simulink model "SlidingModeControl"  (R2018a)
settings: Solver=ode45  StartTime=0.0  StopTime=400  RelTol=1e-3  EnableMultiTasking=on
undefined symbols (not defined in the file or in its folder): sigbuilder_block
libraries: arduino_io_lib x4
settings Model: Creator=Gabriel  LastModifiedBy=Aluno
settings DataIOCC: LimitDataPoints=on  SaveFormat=Array
settings OptimizationCC: LifeSpan=inf
settings DebuggingCC: UnderspecifiedInitializationDetection=Classic  MergeDetectMultiDrivingBlocksExec=none  SolverPrmCheckMsg=warning  StateNameClashWarn=warning  SFUnexpectedBacktrackingDiag=warning  SFNoUnconditionalDefaultTransitionDiag=warning  SFExecutionAtInitializationDiag=none
settings HardwareCC: ProdBitPerPointer=32  ProdBitPerSizeT=32  ProdBitPerPtrDiffT=32  ProdLargestAtomicFloat=None  ProdIntDivRoundTo=Undefined  ProdEndianess=Unspecified  ProdWordSize=32  ProdHWDeviceType=32-bit Generic
settings ModelReferenceCC: PropagateSignalLabelsOutOfModel=off
settings CodeAppCC: StateflowObjectComments=on
settings GRTTargetCC: TargetLangStandard=C89/C90 (ANSI)  GeneratePreprocessorConditionals=Disable all
settings ConfigComp: CovMetricSettings=dw  CovHtmlReporting=on  CovSaveCumulativeToWorkspaceVar=on  CovSaveSingleToWorkspaceVar=on  CovExternalEMLEnable=off

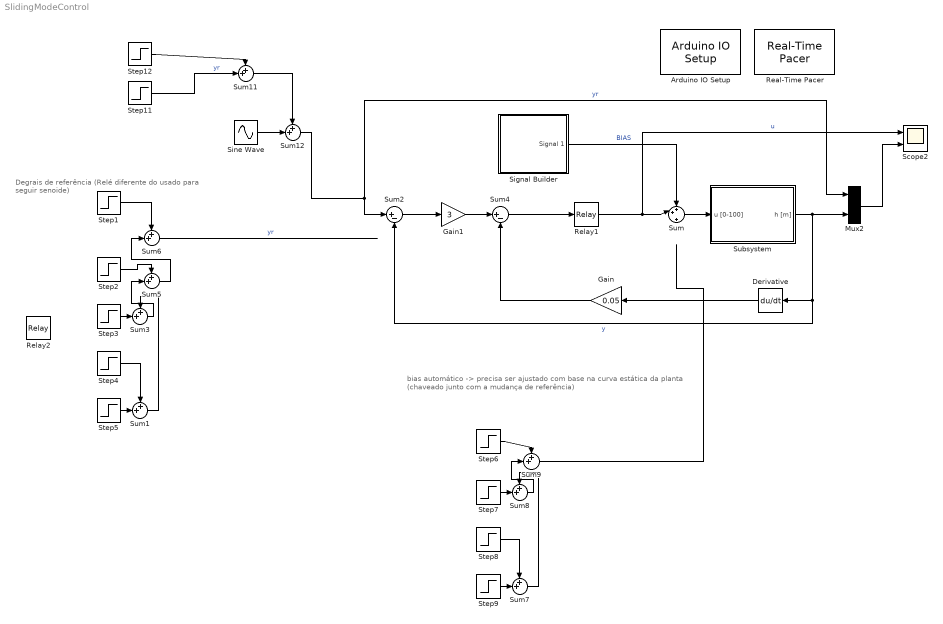
== system SlidingModeControl ==
  note: Degrais de
      | referência
      |
      |
      |
      |
      |
      | (Relé diferente
      | do usado
      | para seguir
      | senoide)
  note: bias automático
      | -> precisa ser ajustado com base na curva estática da planta
      | (chaveado junto com a mudança de referência)
  Arduino IO Setup : arduino_io_lib/Arduino IO Setup  Priority=3  arduinoVar=Temporary arduino variable: Arduino1  workspaceVarName=a  comPort=COM7
  Derivative : Derivative
  Gain : Gain  Gain=0.05
  Gain1 : Gain  Gain=3
  Mux2 : Mux  Inputs=2
  Real-Time Pacer : arduino_io_lib/Real-Time Pacer  simTimePerRealTime=1
  Relay1 : Relay  OffSwitchValue=-eps  OnOutputValue=3
  Relay2 : Relay  OffSwitchValue=-eps  OnOutputValue=1.5
  Scope2 : Scope  NumInputPorts=2
  Signal Builder : Subsystem  Tag=STV Subsys  LoadFcn=sigbuilder_block('load');  StartFcn=sigbuilder_block('start');  StopFcn=sigbuilder_block('stop');  ClipboardFcn=sigbuilder_block('clipboard');  mask(Sigbuilder block){tuvar=[0:10]}
      mask help: Simulink:masks:SigbuilderBlock_MD
      mask init:
      | if ~strcmp(get_param(bdroot(gcbh),'SimulationStatus'),'stopped') tuvar = sigbuilder_block('maskInit'); end
      settings: CopyFcn=sigbuilder_block('copy');  DeleteFcn=sigbuilder_block('delete');  ModelCloseFcn=sigbuilder_block('modelClose');  PreSaveFcn=sigbuilder_block('preSave');  PauseFcn=sigbuilder_block('pause');  ContinueFcn=sigbuilder_block('continue');  NameChangeFcn=sigbuilder_block('namechange');  OpenFcn=sigbuilder_block('open',[6 30 1188 546.75 ]);  CloseFcn=sigbuilder_block('close');
      mask Display: plot(0, 0, 100, 100,[2, 2, 32, 32, 2], [68, 8, 8, 68, 68],[32, 2], [38, 38], [32, 19, 2],[53, 60, 44], [32, 17, 17, 2],[16, 16, 31, 31]);txt = getActiveGroup(gcbh);text(2, 100, txt,'verticalAlignment', 'top');
  Sine Wave : Sin  Amplitude=0.05  Frequency=0.2  SampleTime=0
  Step1 : Step  Time=25  Before=0.6  After=0.55  SampleTime=0
  Step11 : Step  Time=25  Before=0.7  After=0.7  SampleTime=0
  Step12 : Step  Time=0  After=-0.2  SampleTime=0
  Step2 : Step  Time=50  After=0.05  SampleTime=0
  Step3 : Step  Time=75  After=-0.05  SampleTime=0
  Step4 : Step  Time=100  After=-0.05  SampleTime=0
  Step5 : Step  Time=125  After=+0.1  SampleTime=0
  Step6 : Step  Time=50  After=1.5  SampleTime=0
  Step7 : Step  Time=75  After=-1.5  SampleTime=0
  Step8 : Step  Time=100  After=0  SampleTime=0
  Step9 : Step  Time=125  SampleTime=0
  Subsystem : Subsystem
  Sum : Sum  Inputs=++|+
  Sum{1,3,5..9,11..12} (9 alike) : Sum  Inputs=++|
  Sum2 : Sum  Inputs=|+-
  Sum4 : Sum  Inputs=|+-
  wires:
  Subsystem/1(h [m]) -> Mux2/2, Sum2/2, Derivative/1  "y"
  Sum/1 -> Subsystem/1(u [0-100])
  Signal Builder/1(Signal 1) -> Sum/1  "BIAS"
  Gain1/1 -> Sum4/1
  Gain/1 -> Sum4/2
  Sum2/1 -> Gain1/1
  Relay1/1 -> Scope2/1, Sum/2  "u"
  Sum4/1 -> Relay1/1
  Derivative/1 -> Gain/1
  Mux2/1 -> Scope2/2
  Step5/1 -> Sum1/2
  Step4/1 -> Sum1/1
  Sum1/1 -> Sum3/1
  Step3/1 -> Sum3/2
  Sum3/1 -> Sum5/2
  Step2/1 -> Sum5/1
  Step1/1 -> Sum6/1
  Sum5/1 -> Sum6/2
  Sum7/1 -> Sum8/1
  Step8/1 -> Sum7/1
  Sum8/1 -> Sum9/2
  Step7/1 -> Sum8/2
  Step9/1 -> Sum7/2
  Step6/1 -> Sum9/1
  Sum12/1 -> Mux2/1, Sum2/1  "yr"
  Step12/1 -> Sum11/1
  Step11/1 -> Sum11/2  "yr"
  Sum11/1 -> Sum12/1
  Sine Wave/1 -> Sum12/2
  Sum9/1 -> ?
  Sum6/1 -> ?  "yr"

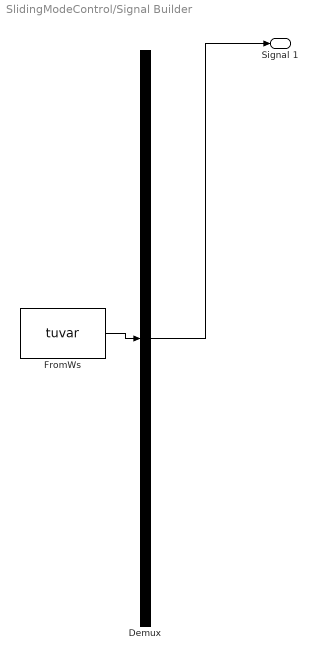
== system SlidingModeControl/Signal Builder ==
  Demux : Demux  Tag=STV Demux  Outputs=1
  FromWs : FromWorkspace  Tag=STV FromWs  VariableName=tuvar  SampleTime=0
      SigBuilderData=|
      | common.afterFinalStr = 'Extrapolate'
      | common.sampleTime = 0
      | dataSet.timeRange = [0 50]
      | dataSet.name = 'Group 1'
      | sbobj.Groups.Name = 'Group 1'
      | sbobj.Groups.Signals.Name = 'Signal 1'
      | sbobj.Groups.Signals.XData = [0 1 1 1.4 1.4 50]
      | sbobj.Groups.Signals.YData = [0 0 74.2 74.2 38.5 38.5]
      | sbobj.Groups.TimeRange = [0 50]
  Signal 1 : Outport  Tag=STV Outport
  wires:
  Demux/1 -> Signal 1/1
  FromWs/1 -> Demux/1

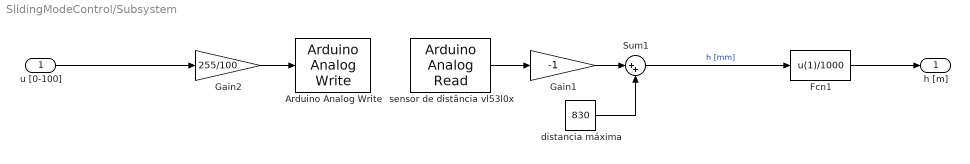
== system SlidingModeControl/Subsystem ==
  u [0-100] : Inport
  Arduino Analog Write : arduino_io_lib/Arduino Analog Write  arduinoVar=Temporary arduino variable: Arduino1  arduinoPin=5  T=0.2
  Fcn1 : Fcn  Expr=u(1)/1000
  Gain1 : Gain  Gain=-1
  Gain2 : Gain  Gain=255/100
  Sum1 : Sum  Inputs=|++
  distancia máxima : Constant  Value=830
  "sensor de distância vl53l0x " : arduino_io_lib/Arduino Analog Read  arduinoVar=Temporary arduino variable: Arduino1  arduinoPin=0  T=0.5
  h [m] : Outport
  wires:
  distancia máxima/1 -> Sum1/2
  Sum1/1 -> Fcn1/1  "h [mm]"
  Gain1/1 -> Sum1/1
  "sensor de distância vl53l0x "/1 -> Gain1/1
  Gain2/1 -> Arduino Analog Write/1
  u [0-100]/1 -> Gain2/1
  Fcn1/1 -> h [m]/1
